simulink model "PFN"  (R2024b)
settings: Solver=daessc  StartTime=0.0  StopTime=0.05  MaxStep=8.0000000000000007E-7  RelTol=1e-3  AbsTol=1e-3
undefined symbols (not defined in the file or in its folder): RCharge, ZLoad
libraries: fl_lib x129, nesl_utility x14
settings Model: Creator=rayri  LastModifiedBy=rayri
settings SolverCC: AlgebraicLoopSolver=TrustRegion  MaxZcPerStep=1
settings DebuggingCC: UnconnectedInputMsg=warning  UnconnectedOutputMsg=warning  UnconnectedLineMsg=warning  SymbolicDimsDataTypeCodeGenerationDiagnostic=none
settings ModelReferenceCC: EnableRefExpFcnMdlSchedulingChecks=on
settings SFSimCC: CustomCodeUndefinedFunction=UseInterfaceOnly
settings RTWCC: GPUComputeCapability=3.5  DLArmComputeVersion=19.05
settings SimscapeCC: SimscapeLogType=all  SimscapeLogSimulationStatistics=on  SimscapeLogDataHistory=10000

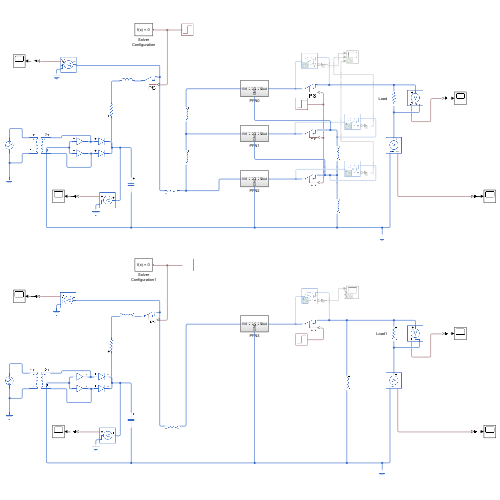
[thumbnail: Simulink's stored preview of the top-level diagram]
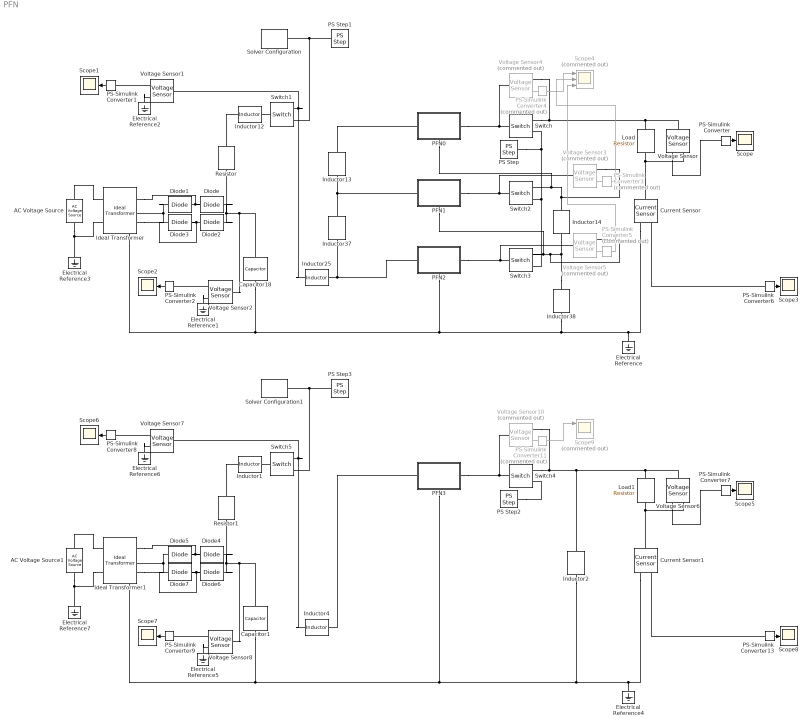
== system PFN ==
  AC Voltage Source : fl_lib/Electrical/Electrical Sources/AC Voltage Source  amp=170 V  shift=0 deg  frequency=60 Hz
  AC Voltage Source1 : fl_lib/Electrical/Electrical Sources/AC Voltage Source  amp=510 V  shift=0 deg  frequency=60 Hz
  Capacitor1 : fl_lib/Electrical/Electrical Elements/Capacitor  c=1e-6 F  r=1e-6 Ohm  g=0 1/Ohm  i_specify=off  i_priority=None  i=0 A  i_nominal_specify=off  i_nominal_value=1  i_nominal_unit=A  v_specify=off  v_priority=None  v=0 V  v_nominal_specify=off  v_nominal_value=1  v_nominal_unit=V  vc_specify=off  vc_priority=High  vc=0 V  vc_nominal_specify=off  vc_nominal_value=1  vc_nominal_unit=V
  Capacitor18 : fl_lib/Electrical/Electrical Elements/Capacitor  c=1e-6 F  r=1e-6 Ohm  g=0 1/Ohm  i_specify=off  i_priority=None  i=0 A  i_nominal_specify=off  i_nominal_value=1  i_nominal_unit=A  v_specify=off  v_priority=None  v=0 V  v_nominal_specify=off  v_nominal_value=1  v_nominal_unit=V  vc_specify=off  vc_priority=High  vc=0 V  vc_nominal_specify=off  vc_nominal_value=1  vc_nominal_unit=V
  Current Sensor : fl_lib/Electrical/Electrical Sensors/Current Sensor
  Current Sensor1 : fl_lib/Electrical/Electrical Sensors/Current Sensor
  Diode{,1..7} (8 alike) : fl_lib/Electrical/Electrical Elements/Diode  Vf=0.6 V  Ron=0.3 Ohm  Goff=1e-8 1/Ohm  i_specify=off  i_priority=None  i=0 A  i_nominal_specify=off  i_nominal_value=1  i_nominal_unit=A  v_specify=off  v_priority=None  v=0 V  v_nominal_specify=off  v_nominal_value=1  v_nominal_unit=V
  Electrical Reference{,1..7} (8 alike) : fl_lib/Electrical/Electrical Elements/Electrical Reference
  Ideal Transformer : fl_lib/Electrical/Electrical Elements/Ideal Transformer  n=0.25  i1_specify=off  i1_priority=None  i1=0 A  i1_nominal_specify=off  i1_nominal_value=1  i1_nominal_unit=A  v1_specify=off  v1_priority=None  v1=0 V  v1_nominal_specify=off  v1_nominal_value=1  v1_nominal_unit=V  i2_specify=off  i2_priority=None  i2=0 A  i2_nominal_specify=off  i2_nominal_value=1  i2_nominal_unit=A  v2_specify=off  v2_priority=None  v2=0 V  v2_nominal_specify=off  v2_nominal_value=1  v2_nominal_unit=V
  Ideal Transformer1 : fl_lib/Electrical/Electrical Elements/Ideal Transformer  n=0.25  i1_specify=off  i1_priority=None  i1=0 A  i1_nominal_specify=off  i1_nominal_value=1  i1_nominal_unit=A  v1_specify=off  v1_priority=None  v1=0 V  v1_nominal_specify=off  v1_nominal_value=1  v1_nominal_unit=V  i2_specify=off  i2_priority=None  i2=0 A  i2_nominal_specify=off  i2_nominal_value=1  i2_nominal_unit=A  v2_specify=off  v2_priority=None  v2=0 V  v2_nominal_specify=off  v2_nominal_value=1  v2_nominal_unit=V
  Inductor{1..2,4,12..14,25,37..38} (9 alike) : fl_lib/Electrical/Electrical Elements/Inductor  l=LIso H  r=1e-3 Ohm  g=1e-9 1/Ohm  i_specify=off  i_priority=None  i=0 A  i_nominal_specify=off  i_nominal_value=1  i_nominal_unit=A  v_specify=off  v_priority=None  v=0 V  v_nominal_specify=off  v_nominal_value=1  v_nominal_unit=V  i_L_specify=off  i_L_priority=High  i_L=0 A  i_L_nominal_specify=off  i_L_nominal_value=1  i_L_nominal_unit=A
  Load : fl_lib/Electrical/Electrical Elements/Resistor  R=ZLoad Ohm  i_specify=off  i_priority=None  i=0 A  i_nominal_specify=off  i_nominal_value=1  i_nominal_unit=A  v_specify=off  v_priority=None  v=0 V  v_nominal_specify=off  v_nominal_value=1  v_nominal_unit=V
  Load1 : fl_lib/Electrical/Electrical Elements/Resistor  R=ZLoad Ohm  i_specify=off  i_priority=None  i=0 A  i_nominal_specify=off  i_nominal_value=1  i_nominal_unit=A  v_specify=off  v_priority=None  v=0 V  v_nominal_specify=off  v_nominal_value=1  v_nominal_unit=V
  PFN0 : Subsystem
      settings: PortSchema="{\"entries\":[{\"content\":{\"sides\":[{\"content\":{\"connectorIds\":[\"LConn1\"]},\"type\":\"ConnectorPlacement.EquallySpacedRectSide\",\"uuid\":\"fdd4c1f4-74f1-49d2-92a3-a8a9509127e0\"},{\"content\":{\"connectorIds\":[\"RConn1\"],\"side\":\"RIGHT\"},\"type\":\"ConnectorPlacement.EquallySpacedRectSide\",\"uuid\":\"4868eeaf-41c4-4471-80cb-0808ac67c1cc\"},{\"content\":{\"side\":\"TOP\"},\"type\":\"ConnectorPlacement.EquallySpacedRectSide\",\"uuid\":\"1036f9ad-0bf3-475a-a2be-7d60f94794c2\"},{\"content\":{\"connectorIds\":[\"RConn2\"],\"side\":\"BOTTOM\"},\"type\":\"ConnectorPlacement.EquallySpacedRectSide\",\"uuid\":\"b0e9804a-444c-47a9-aebb-e44828666ae9\"}]},\"type\":\"ConnectorPlacement.EquallySpacedConnector\",\"uuid\":\"dcb91c64-926f-48f4-8d63-1ba7813f4e16\"}],\"packageUris\":[\"http://schema.mathworks.com/mf0/Connector/R2020b\"],\"version\":\"1.0\"}"
  PFN1 : Subsystem
      settings: PortSchema="{\"entries\":[{\"content\":{\"sides\":[{\"content\":{\"connectorIds\":[\"LConn1\"]},\"type\":\"ConnectorPlacement.EquallySpacedRectSide\",\"uuid\":\"fdd4c1f4-74f1-49d2-92a3-a8a9509127e0\"},{\"content\":{\"connectorIds\":[\"RConn1\"],\"side\":\"RIGHT\"},\"type\":\"ConnectorPlacement.EquallySpacedRectSide\",\"uuid\":\"4868eeaf-41c4-4471-80cb-0808ac67c1cc\"},{\"content\":{\"side\":\"TOP\"},\"type\":\"ConnectorPlacement.EquallySpacedRectSide\",\"uuid\":\"1036f9ad-0bf3-475a-a2be-7d60f94794c2\"},{\"content\":{\"connectorIds\":[\"RConn2\"],\"side\":\"BOTTOM\"},\"type\":\"ConnectorPlacement.EquallySpacedRectSide\",\"uuid\":\"b0e9804a-444c-47a9-aebb-e44828666ae9\"}]},\"type\":\"ConnectorPlacement.EquallySpacedConnector\",\"uuid\":\"dcb91c64-926f-48f4-8d63-1ba7813f4e16\"}],\"packageUris\":[\"http://schema.mathworks.com/mf0/Connector/R2020b\"],\"version\":\"1.0\"}"
  PFN2 : Subsystem
      settings: PortSchema="{\"entries\":[{\"content\":{\"sides\":[{\"content\":{\"connectorIds\":[\"LConn1\"]},\"type\":\"ConnectorPlacement.EquallySpacedRectSide\",\"uuid\":\"fdd4c1f4-74f1-49d2-92a3-a8a9509127e0\"},{\"content\":{\"connectorIds\":[\"RConn1\"],\"side\":\"RIGHT\"},\"type\":\"ConnectorPlacement.EquallySpacedRectSide\",\"uuid\":\"4868eeaf-41c4-4471-80cb-0808ac67c1cc\"},{\"content\":{\"side\":\"TOP\"},\"type\":\"ConnectorPlacement.EquallySpacedRectSide\",\"uuid\":\"1036f9ad-0bf3-475a-a2be-7d60f94794c2\"},{\"content\":{\"connectorIds\":[\"RConn2\"],\"side\":\"BOTTOM\"},\"type\":\"ConnectorPlacement.EquallySpacedRectSide\",\"uuid\":\"b0e9804a-444c-47a9-aebb-e44828666ae9\"}]},\"type\":\"ConnectorPlacement.EquallySpacedConnector\",\"uuid\":\"dcb91c64-926f-48f4-8d63-1ba7813f4e16\"}],\"packageUris\":[\"http://schema.mathworks.com/mf0/Connector/R2020b\"],\"version\":\"1.0\"}"
  PFN3 : Subsystem
      settings: PortSchema="{\"entries\":[{\"content\":{\"sides\":[{\"content\":{\"connectorIds\":[\"LConn1\"]},\"type\":\"ConnectorPlacement.EquallySpacedRectSide\",\"uuid\":\"fdd4c1f4-74f1-49d2-92a3-a8a9509127e0\"},{\"content\":{\"connectorIds\":[\"RConn1\"],\"side\":\"RIGHT\"},\"type\":\"ConnectorPlacement.EquallySpacedRectSide\",\"uuid\":\"4868eeaf-41c4-4471-80cb-0808ac67c1cc\"},{\"content\":{\"side\":\"TOP\"},\"type\":\"ConnectorPlacement.EquallySpacedRectSide\",\"uuid\":\"1036f9ad-0bf3-475a-a2be-7d60f94794c2\"},{\"content\":{\"connectorIds\":[\"RConn2\"],\"side\":\"BOTTOM\"},\"type\":\"ConnectorPlacement.EquallySpacedRectSide\",\"uuid\":\"b0e9804a-444c-47a9-aebb-e44828666ae9\"}]},\"type\":\"ConnectorPlacement.EquallySpacedConnector\",\"uuid\":\"dcb91c64-926f-48f4-8d63-1ba7813f4e16\"}],\"packageUris\":[\"http://schema.mathworks.com/mf0/Connector/R2020b\"],\"version\":\"1.0\"}"
  PS Step : fl_lib/Physical Signals/Sources/PS Step  step_time=0.02 s  initial_value=0  final_value=1
  PS Step1 : fl_lib/Physical Signals/Sources/PS Step  step_time=0.01 s  initial_value=1  final_value=0
  PS Step2 : fl_lib/Physical Signals/Sources/PS Step  step_time=0.02 s  initial_value=0  final_value=1
  PS Step3 : fl_lib/Physical Signals/Sources/PS Step  step_time=0.01 s  initial_value=1  final_value=0
  PS-Simulink Converter{,1..2,6..9,13} (8 alike) : nesl_utility/PS-Simulink Converter  PhysicalDomain=network_engine_domain  SubClassName=ps_output  LeftPortType=input  RightPortType=output  PseudoPeriodic=off  Frequencies=[]  VectorFormat=inherit  Unit=inherit  AffineConversion=off
  PS-Simulink Converter{3..5,11} (4 alike) : nesl_utility/PS-Simulink Converter  Commented=on  PhysicalDomain=network_engine_domain  SubClassName=ps_output  LeftPortType=input  RightPortType=output  PseudoPeriodic=off  Frequencies=[]  VectorFormat=inherit  Unit=inherit  AffineConversion=off
  Resistor : fl_lib/Electrical/Electrical Elements/Resistor  R=RCharge Ohm  i_specify=off  i_priority=None  i=0 A  i_nominal_specify=off  i_nominal_value=1  i_nominal_unit=A  v_specify=off  v_priority=None  v=0 V  v_nominal_specify=off  v_nominal_value=1  v_nominal_unit=V
  Resistor1 : fl_lib/Electrical/Electrical Elements/Resistor  R=RCharge Ohm  i_specify=off  i_priority=None  i=0 A  i_nominal_specify=off  i_nominal_value=1  i_nominal_unit=A  v_specify=off  v_priority=None  v=0 V  v_nominal_specify=off  v_nominal_value=1  v_nominal_unit=V
  Scope{,1..3,5..8} (8 alike) : Scope
  Scope4 : Scope  Commented=on  NumInputPorts=3
  Scope9 : Scope  Commented=on  NumInputPorts=3
  Solver Configuration : nesl_utility/Solver Configuration  PhysicalDomain=network_engine_domain  SubClassName=solver  LeftPortType=input  RightPortType=generic  Tones=[]  Harmonics=[]  SimulateNoise=off  Profile=off  UseLocalSampling=off  EnableSwitchedLinearOptims=on  FrequencyDomain=off  UseCCode=off  RelTol=0.001  AbsTol=1e-06  MinStep=1e-09  ToWorkspace=off  RevertToSquareIcSolve=off  NumHomotopyIterations=100  PhasorMode=off  PhasorModeNumHarmonics=1  ConsistencySolver=NEWTON_XTOL_AFTER_FTOL  IndexReductionMethod=Projection  DoDC=off  ResidualTolerance=1e-09  ConsistencyTolSource=GLOBAL  ConsistencyAbsTol=0.001  ConsistencyRelTol=0.001  ConsistencyTolFactor=0.001  UseLocalSolver=off  LocalSolverChoice=NE_BACKWARD_EULER_ADVANCER  ResolveIndetEquations=on  FunctionEvalNumThread=1  LocalSolverSampleTime=0.001  DoFixedCost=off  MaxNonlinIter=3  MaxModeIter=2  ComputeImpulses=off  ImpulseIterations=2  LinearAlgebra=auto  LinearAlgebraNumThread=0  EquationFormulation=NE_TIME_EF  DelaysMemoryBudget=1024  AutomaticFiltering=on  FilteringTimeConstant=0.001  PartitionStorageMethod=AS_NEEDED  PartitionMemoryBudget=1024  PartitionMethod=ROBUST  MultibodyUseLocalSolver=off  MultibodyLocalSolverChoice=ODE1  MultibodyLocalSolverSampleTime=0.001
  Solver Configuration1 : nesl_utility/Solver Configuration  PhysicalDomain=network_engine_domain  SubClassName=solver  LeftPortType=input  RightPortType=generic  Tones=[]  Harmonics=[]  SimulateNoise=off  Profile=off  UseLocalSampling=off  EnableSwitchedLinearOptims=on  FrequencyDomain=off  UseCCode=off  RelTol=0.001  AbsTol=1e-06  MinStep=1e-09  ToWorkspace=off  RevertToSquareIcSolve=off  NumHomotopyIterations=100  PhasorMode=off  PhasorModeNumHarmonics=1  ConsistencySolver=NEWTON_XTOL_AFTER_FTOL  IndexReductionMethod=Projection  DoDC=off  ResidualTolerance=1e-09  ConsistencyTolSource=GLOBAL  ConsistencyAbsTol=0.001  ConsistencyRelTol=0.001  ConsistencyTolFactor=0.001  UseLocalSolver=off  LocalSolverChoice=NE_BACKWARD_EULER_ADVANCER  ResolveIndetEquations=on  FunctionEvalNumThread=1  LocalSolverSampleTime=0.001  DoFixedCost=off  MaxNonlinIter=3  MaxModeIter=2  ComputeImpulses=off  ImpulseIterations=2  LinearAlgebra=auto  LinearAlgebraNumThread=0  EquationFormulation=NE_TIME_EF  DelaysMemoryBudget=1024  AutomaticFiltering=on  FilteringTimeConstant=0.001  PartitionStorageMethod=AS_NEEDED  PartitionMemoryBudget=1024  PartitionMethod=ROBUST  MultibodyUseLocalSolver=off  MultibodyLocalSolverChoice=ODE1  MultibodyLocalSolverSampleTime=0.001
  Switch{,1..5} (6 alike) : fl_lib/Electrical/Electrical Elements/Switch  R_closed=0.01 Ohm  G_open=1e-8 1/Ohm  Threshold=0.5  i_specify=off  i_priority=None  i=0 A  i_nominal_specify=off  i_nominal_value=1  i_nominal_unit=A  v_specify=off  v_priority=None  v=0 V  v_nominal_specify=off  v_nominal_value=1  v_nominal_unit=V
  Voltage Sensor{,1..2,6..8} (6 alike) : fl_lib/Electrical/Electrical Sensors/Voltage Sensor
  Voltage Sensor{3..5,10} (4 alike) : fl_lib/Electrical/Electrical Sensors/Voltage Sensor  Commented=on
  wires:
  PS-Simulink Converter/1 -> Scope/1
  PS-Simulink Converter1/1 -> Scope1/1
  PS-Simulink Converter2/1 -> Scope2/1
  PS-Simulink Converter4/1 -> Scope4/1
  PS-Simulink Converter3/1 -> Scope4/2
  PS-Simulink Converter5/1 -> Scope4/3
  PS-Simulink Converter6/1 -> Scope3/1
  PS-Simulink Converter13/1 -> Scope8/1
  PS-Simulink Converter8/1 -> Scope6/1
  PS-Simulink Converter11/1 -> Scope9/1
  PS-Simulink Converter7/1 -> Scope5/1
  PS-Simulink Converter9/1 -> Scope7/1
  connections:
  PS Step/RConn1 -- Switch/RConn1 -- Switch3/RConn1 -- Switch2/RConn1
  Voltage Sensor/LConn1 -- Voltage Sensor4/RConn2 -- Switch/RConn2 -- Load/LConn1
  Voltage Sensor/RConn1 -- PS-Simulink Converter/LConn1
  PS Step1/RConn1 -- Switch1/RConn1 -- Solver Configuration/RConn1
  Voltage Sensor1/RConn1 -- PS-Simulink Converter1/LConn1
  Inductor37/LConn1 -- PFN1/LConn1 -- Inductor13/RConn1
  PFN1/RConn1 -- Voltage Sensor3/LConn1 -- Switch2/LConn1
  Diode1/LConn1 -- Capacitor18/RConn1 -- PFN2/RConn2 -- Current Sensor/RConn2 -- Electrical Reference/LConn1 -- Inductor38/RConn1 -- Diode3/LConn1
  Switch2/RConn2 -- PFN0/RConn2 -- Voltage Sensor3/RConn2 -- Inductor14/LConn1
  Inductor12/LConn1 -- Resistor/RConn1
  Inductor12/RConn1 -- Switch1/LConn1
  Diode/RConn1 -- Capacitor18/LConn1 -- Voltage Sensor2/LConn1 -- Resistor/LConn1 -- Diode2/RConn1
  Switch1/RConn2 -- Inductor25/RConn1 -- Voltage Sensor1/LConn1
  Inductor25/LConn1 -- PFN2/LConn1 -- Inductor37/RConn1
  PFN2/RConn1 -- Voltage Sensor5/LConn1 -- Switch3/LConn1
  Diode1/RConn1 -- Ideal Transformer/RConn1 -- Diode/LConn1
  Diode2/LConn1 -- Ideal Transformer/RConn2 -- Diode3/RConn1
  Electrical Reference2/LConn1 -- Voltage Sensor1/RConn2
  PFN0/RConn1 -- Voltage Sensor4/LConn1 -- Switch/LConn1
  PFN0/LConn1 -- Inductor13/LConn1
  Inductor38/LConn1 -- Voltage Sensor5/RConn2 -- PFN1/RConn2 -- Switch3/RConn2 -- Inductor14/RConn1
  Voltage Sensor2/RConn1 -- PS-Simulink Converter2/LConn1
  Electrical Reference1/LConn1 -- Voltage Sensor2/RConn2
  AC Voltage Source/RConn1 -- Electrical Reference3/LConn1 -- Ideal Transformer/LConn2
  AC Voltage Source/LConn1 -- Ideal Transformer/LConn1
  PS-Simulink Converter4/LConn1 -- Voltage Sensor4/RConn1
  PS-Simulink Converter3/LConn1 -- Voltage Sensor3/RConn1
  PS-Simulink Converter5/LConn1 -- Voltage Sensor5/RConn1
  Load/RConn1 -- Current Sensor/LConn1 -- Voltage Sensor/RConn2
  PS-Simulink Converter6/LConn1 -- Current Sensor/RConn1
  Load1/RConn1 -- Current Sensor1/LConn1 -- Voltage Sensor6/RConn2
  PFN3/LConn1 -- Inductor4/LConn1
  Electrical Reference4/LConn1 -- Current Sensor1/RConn2 -- Inductor2/RConn1 -- PFN3/RConn2 -- Diode7/LConn1 -- Diode5/LConn1 -- Capacitor1/RConn1
  Switch4/RConn2 -- Voltage Sensor10/RConn2 -- Inductor2/LConn1 -- Voltage Sensor6/LConn1 -- Load1/LConn1
  Solver Configuration1/RConn1 -- PS Step3/RConn1 -- Switch5/RConn1
  Diode6/RConn1 -- Diode4/RConn1 -- Capacitor1/LConn1 -- Voltage Sensor8/LConn1 -- Resistor1/LConn1
  Ideal Transformer1/LConn2 -- AC Voltage Source1/RConn1 -- Electrical Reference7/LConn1
  Diode4/LConn1 -- Diode5/RConn1 -- Ideal Transformer1/RConn1
  Switch4/LConn1 -- PFN3/RConn1 -- Voltage Sensor10/LConn1
  PS Step2/RConn1 -- Switch4/RConn1
  Diode7/RConn1 -- Diode6/LConn1 -- Ideal Transformer1/RConn2
  Voltage Sensor7/LConn1 -- Switch5/RConn2 -- Inductor4/RConn1
  AC Voltage Source1/LConn1 -- Ideal Transformer1/LConn1
  PS-Simulink Converter11/LConn1 -- Voltage Sensor10/RConn1
  Voltage Sensor7/RConn1 -- PS-Simulink Converter8/LConn1
  Electrical Reference6/LConn1 -- Voltage Sensor7/RConn2
  Inductor1/LConn1 -- Resistor1/RConn1
  Inductor1/RConn1 -- Switch5/LConn1
  Voltage Sensor6/RConn1 -- PS-Simulink Converter7/LConn1
  Voltage Sensor8/RConn1 -- PS-Simulink Converter9/LConn1
  Electrical Reference5/LConn1 -- Voltage Sensor8/RConn2
  PS-Simulink Converter13/LConn1 -- Current Sensor1/RConn1

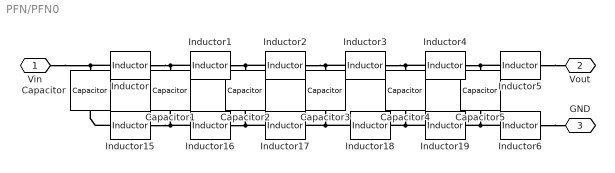
== system PFN/PFN0 ==
  Capacitor{,1..5} (6 alike) : fl_lib/Electrical/Electrical Elements/Capacitor  c=C0 F  r=1e-6 Ohm  g=0 1/Ohm  i_specify=off  i_priority=None  i=0 A  i_nominal_specify=off  i_nominal_value=1  i_nominal_unit=A  v_specify=off  v_priority=None  v=1000 V  v_nominal_specify=off  v_nominal_value=1  v_nominal_unit=V  vc_specify=off  vc_priority=High  vc=1000 V  vc_nominal_specify=off  vc_nominal_value=1  vc_nominal_unit=V
  Inductor{,1..4,6,15..19} (11 alike) : fl_lib/Electrical/Electrical Elements/Inductor  l=L0 H  r=1e-3 Ohm  g=1e-9 1/Ohm  i_specify=off  i_priority=None  i=0 A  i_nominal_specify=off  i_nominal_value=1  i_nominal_unit=A  v_specify=off  v_priority=None  v=0 V  v_nominal_specify=off  v_nominal_value=1  v_nominal_unit=V  i_L_specify=off  i_L_priority=High  i_L=0 A  i_L_nominal_specify=off  i_L_nominal_value=1  i_L_nominal_unit=A
  Inductor5 : fl_lib/Electrical/Electrical Elements/Inductor  l=LTerm H  r=1e-3 Ohm  g=1e-9 1/Ohm  i_specify=off  i_priority=None  i=0 A  i_nominal_specify=off  i_nominal_value=1  i_nominal_unit=A  v_specify=off  v_priority=None  v=0 V  v_nominal_specify=off  v_nominal_value=1  v_nominal_unit=V  i_L_specify=off  i_L_priority=High  i_L=0 A  i_L_nominal_specify=off  i_L_nominal_value=1  i_L_nominal_unit=A
  Vin : PMIOPort  Side=Left
  Vout : PMIOPort  Port=2  Side=Right
  GND : PMIOPort  Port=3  Side=Right
  connections:
  Inductor16/RConn1 -- Inductor17/LConn1 -- Capacitor2/RConn1
  Inductor15/LConn1 -- Capacitor/RConn1
  Capacitor4/RConn1 -- Inductor19/LConn1 -- Inductor18/RConn1
  Capacitor3/RConn1 -- Inductor18/LConn1 -- Inductor17/RConn1
  Inductor5/RConn1 -- Vout/RConn1
  Inductor1/LConn1 -- Inductor/RConn1 -- Capacitor1/LConn1
  Inductor5/LConn1 -- Inductor4/RConn1 -- Capacitor5/LConn1
  Inductor4/LConn1 -- Inductor3/RConn1 -- Capacitor4/LConn1
  Inductor2/LConn1 -- Inductor1/RConn1 -- Capacitor2/LConn1
  Inductor15/RConn1 -- Inductor16/LConn1 -- Capacitor1/RConn1
  Inductor/LConn1 -- Vin/RConn1 -- Capacitor/LConn1
  Inductor19/RConn1 -- Capacitor5/RConn1 -- Inductor6/LConn1
  Inductor3/LConn1 -- Inductor2/RConn1 -- Capacitor3/LConn1
  Inductor6/RConn1 -- GND/RConn1

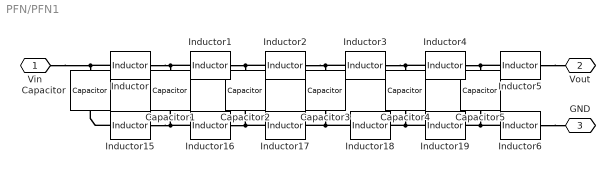
== system PFN/PFN1 ==
  Capacitor{,1..5} (6 alike) : fl_lib/Electrical/Electrical Elements/Capacitor  c=C0 F  r=1e-6 Ohm  g=0 1/Ohm  i_specify=off  i_priority=None  i=0 A  i_nominal_specify=off  i_nominal_value=1  i_nominal_unit=A  v_specify=off  v_priority=None  v=1000 V  v_nominal_specify=off  v_nominal_value=1  v_nominal_unit=V  vc_specify=off  vc_priority=High  vc=1000 V  vc_nominal_specify=off  vc_nominal_value=1  vc_nominal_unit=V
  Inductor{,1..4,6,15..19} (11 alike) : fl_lib/Electrical/Electrical Elements/Inductor  l=L0 H  r=1e-3 Ohm  g=1e-9 1/Ohm  i_specify=off  i_priority=None  i=0 A  i_nominal_specify=off  i_nominal_value=1  i_nominal_unit=A  v_specify=off  v_priority=None  v=0 V  v_nominal_specify=off  v_nominal_value=1  v_nominal_unit=V  i_L_specify=off  i_L_priority=High  i_L=0 A  i_L_nominal_specify=off  i_L_nominal_value=1  i_L_nominal_unit=A
  Inductor5 : fl_lib/Electrical/Electrical Elements/Inductor  l=LTerm H  r=1e-3 Ohm  g=1e-9 1/Ohm  i_specify=off  i_priority=None  i=0 A  i_nominal_specify=off  i_nominal_value=1  i_nominal_unit=A  v_specify=off  v_priority=None  v=0 V  v_nominal_specify=off  v_nominal_value=1  v_nominal_unit=V  i_L_specify=off  i_L_priority=High  i_L=0 A  i_L_nominal_specify=off  i_L_nominal_value=1  i_L_nominal_unit=A
  Vin : PMIOPort  Side=Left
  Vout : PMIOPort  Port=2  Side=Right
  GND : PMIOPort  Port=3  Side=Right
  connections:
  Inductor16/RConn1 -- Inductor17/LConn1 -- Capacitor2/RConn1
  Inductor15/LConn1 -- Capacitor/RConn1
  Capacitor4/RConn1 -- Inductor19/LConn1 -- Inductor18/RConn1
  Capacitor3/RConn1 -- Inductor18/LConn1 -- Inductor17/RConn1
  Inductor5/RConn1 -- Vout/RConn1
  Inductor1/LConn1 -- Inductor/RConn1 -- Capacitor1/LConn1
  Inductor5/LConn1 -- Inductor4/RConn1 -- Capacitor5/LConn1
  Inductor4/LConn1 -- Inductor3/RConn1 -- Capacitor4/LConn1
  Inductor2/LConn1 -- Inductor1/RConn1 -- Capacitor2/LConn1
  Inductor15/RConn1 -- Inductor16/LConn1 -- Capacitor1/RConn1
  Inductor/LConn1 -- Vin/RConn1 -- Capacitor/LConn1
  Inductor19/RConn1 -- Capacitor5/RConn1 -- Inductor6/LConn1
  Inductor3/LConn1 -- Inductor2/RConn1 -- Capacitor3/LConn1
  Inductor6/RConn1 -- GND/RConn1

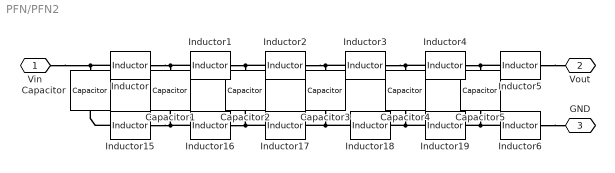
== system PFN/PFN2 ==
  Capacitor{,1..5} (6 alike) : fl_lib/Electrical/Electrical Elements/Capacitor  c=C0 F  r=1e-6 Ohm  g=0 1/Ohm  i_specify=off  i_priority=None  i=0 A  i_nominal_specify=off  i_nominal_value=1  i_nominal_unit=A  v_specify=off  v_priority=None  v=1000 V  v_nominal_specify=off  v_nominal_value=1  v_nominal_unit=V  vc_specify=off  vc_priority=High  vc=1000 V  vc_nominal_specify=off  vc_nominal_value=1  vc_nominal_unit=V
  Inductor{,1..4,6,15..19} (11 alike) : fl_lib/Electrical/Electrical Elements/Inductor  l=L0 H  r=1e-3 Ohm  g=1e-9 1/Ohm  i_specify=off  i_priority=None  i=0 A  i_nominal_specify=off  i_nominal_value=1  i_nominal_unit=A  v_specify=off  v_priority=None  v=0 V  v_nominal_specify=off  v_nominal_value=1  v_nominal_unit=V  i_L_specify=off  i_L_priority=High  i_L=0 A  i_L_nominal_specify=off  i_L_nominal_value=1  i_L_nominal_unit=A
  Inductor5 : fl_lib/Electrical/Electrical Elements/Inductor  l=LTerm H  r=1e-3 Ohm  g=1e-9 1/Ohm  i_specify=off  i_priority=None  i=0 A  i_nominal_specify=off  i_nominal_value=1  i_nominal_unit=A  v_specify=off  v_priority=None  v=0 V  v_nominal_specify=off  v_nominal_value=1  v_nominal_unit=V  i_L_specify=off  i_L_priority=High  i_L=0 A  i_L_nominal_specify=off  i_L_nominal_value=1  i_L_nominal_unit=A
  Vin : PMIOPort  Side=Left
  Vout : PMIOPort  Port=2  Side=Right
  GND : PMIOPort  Port=3  Side=Right
  connections:
  Inductor16/RConn1 -- Inductor17/LConn1 -- Capacitor2/RConn1
  Inductor15/LConn1 -- Capacitor/RConn1
  Capacitor4/RConn1 -- Inductor19/LConn1 -- Inductor18/RConn1
  Capacitor3/RConn1 -- Inductor18/LConn1 -- Inductor17/RConn1
  Inductor5/RConn1 -- Vout/RConn1
  Inductor1/LConn1 -- Inductor/RConn1 -- Capacitor1/LConn1
  Inductor5/LConn1 -- Inductor4/RConn1 -- Capacitor5/LConn1
  Inductor4/LConn1 -- Inductor3/RConn1 -- Capacitor4/LConn1
  Inductor2/LConn1 -- Inductor1/RConn1 -- Capacitor2/LConn1
  Inductor15/RConn1 -- Inductor16/LConn1 -- Capacitor1/RConn1
  Inductor/LConn1 -- Vin/RConn1 -- Capacitor/LConn1
  Inductor19/RConn1 -- Capacitor5/RConn1 -- Inductor6/LConn1
  Inductor3/LConn1 -- Inductor2/RConn1 -- Capacitor3/LConn1
  Inductor6/RConn1 -- GND/RConn1

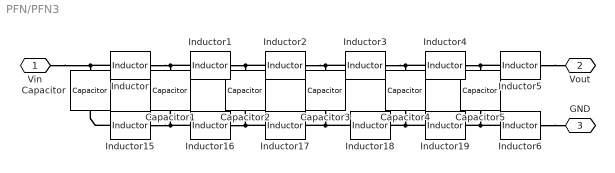
== system PFN/PFN3 ==
  Capacitor{,1..5} (6 alike) : fl_lib/Electrical/Electrical Elements/Capacitor  c=C0 F  r=1e-6 Ohm  g=0 1/Ohm  i_specify=off  i_priority=None  i=0 A  i_nominal_specify=off  i_nominal_value=1  i_nominal_unit=A  v_specify=off  v_priority=None  v=1000 V  v_nominal_specify=off  v_nominal_value=1  v_nominal_unit=V  vc_specify=off  vc_priority=High  vc=1000 V  vc_nominal_specify=off  vc_nominal_value=1  vc_nominal_unit=V
  Inductor{,1..4,6,15..19} (11 alike) : fl_lib/Electrical/Electrical Elements/Inductor  l=L0 H  r=1e-3 Ohm  g=1e-9 1/Ohm  i_specify=off  i_priority=None  i=0 A  i_nominal_specify=off  i_nominal_value=1  i_nominal_unit=A  v_specify=off  v_priority=None  v=0 V  v_nominal_specify=off  v_nominal_value=1  v_nominal_unit=V  i_L_specify=off  i_L_priority=High  i_L=0 A  i_L_nominal_specify=off  i_L_nominal_value=1  i_L_nominal_unit=A
  Inductor5 : fl_lib/Electrical/Electrical Elements/Inductor  l=LTerm H  r=1e-3 Ohm  g=1e-9 1/Ohm  i_specify=off  i_priority=None  i=0 A  i_nominal_specify=off  i_nominal_value=1  i_nominal_unit=A  v_specify=off  v_priority=None  v=0 V  v_nominal_specify=off  v_nominal_value=1  v_nominal_unit=V  i_L_specify=off  i_L_priority=High  i_L=0 A  i_L_nominal_specify=off  i_L_nominal_value=1  i_L_nominal_unit=A
  Vin : PMIOPort  Side=Left
  Vout : PMIOPort  Port=2  Side=Right
  GND : PMIOPort  Port=3  Side=Right
  connections:
  Inductor16/RConn1 -- Inductor17/LConn1 -- Capacitor2/RConn1
  Inductor15/LConn1 -- Capacitor/RConn1
  Capacitor4/RConn1 -- Inductor19/LConn1 -- Inductor18/RConn1
  Capacitor3/RConn1 -- Inductor18/LConn1 -- Inductor17/RConn1
  Inductor5/RConn1 -- Vout/RConn1
  Inductor1/LConn1 -- Inductor/RConn1 -- Capacitor1/LConn1
  Inductor5/LConn1 -- Inductor4/RConn1 -- Capacitor5/LConn1
  Inductor4/LConn1 -- Inductor3/RConn1 -- Capacitor4/LConn1
  Inductor2/LConn1 -- Inductor1/RConn1 -- Capacitor2/LConn1
  Inductor15/RConn1 -- Inductor16/LConn1 -- Capacitor1/RConn1
  Inductor/LConn1 -- Vin/RConn1 -- Capacitor/LConn1
  Inductor19/RConn1 -- Capacitor5/RConn1 -- Inductor6/LConn1
  Inductor3/LConn1 -- Inductor2/RConn1 -- Capacitor3/LConn1
  Inductor6/RConn1 -- GND/RConn1
